simulink model "assignment_12_impedance_control_2022a"  (R2022a)
settings: Solver=VariableStepAuto  StartTime=0.0  StopTime=10  RelTol=1e-3
values from neighbouring files (symbols this model uses):
  dq0 = [0;0;0]    [assignment_10.m]    (also in assignment_11.m; assignment_12.m; assignment_13.m; assignment_6.m)
  K_env = 1000    [assignment_11.m]    (also in assignment_12.m = 100; assignment_13.m = 100)
  Kd = 100    [assignment_10.m]    (also in assignment_11.m = 1000; assignment_12.m; assignment_6.m = 1000; assignment_7.m = diag(2 * xi .* w))
  Kp = 1000    [assignment_10.m]    (also in assignment_11.m = 10000; assignment_12.m; assignment_6.m; assignment_7.m = diag(w .* w))
  q0 = [0;0;0]    [assignment_10.m]    (also in assignment_11.m; assignment_12.m; assignment_13.m = [0; pi/2; -pi/2]; assignment_6.m)
  traj = [q1_d; q2_d; q3_d]    [assignment_10.m]    (also in assignment_12.m; assignment_7.m)
  x_rest_env = direct_kinematics(q_rest_env)    [assignment_11.m]    (also in assignment_12.m; assignment_13.m = x_rest_env(1:3, 1))
libraries: robotcorelib x1
settings Model: Creator=acesi  LastModifiedBy=Manu
settings ModelReferenceCC: EnableRefExpFcnMdlSchedulingChecks=off
settings RTWCC: Description=Generic Real-Time Target

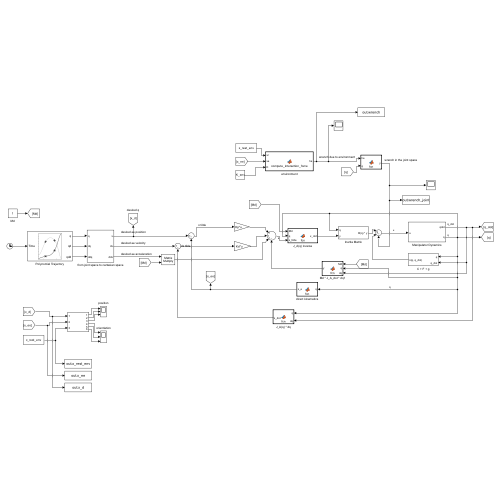
[thumbnail: Simulink's stored preview of the top-level diagram]
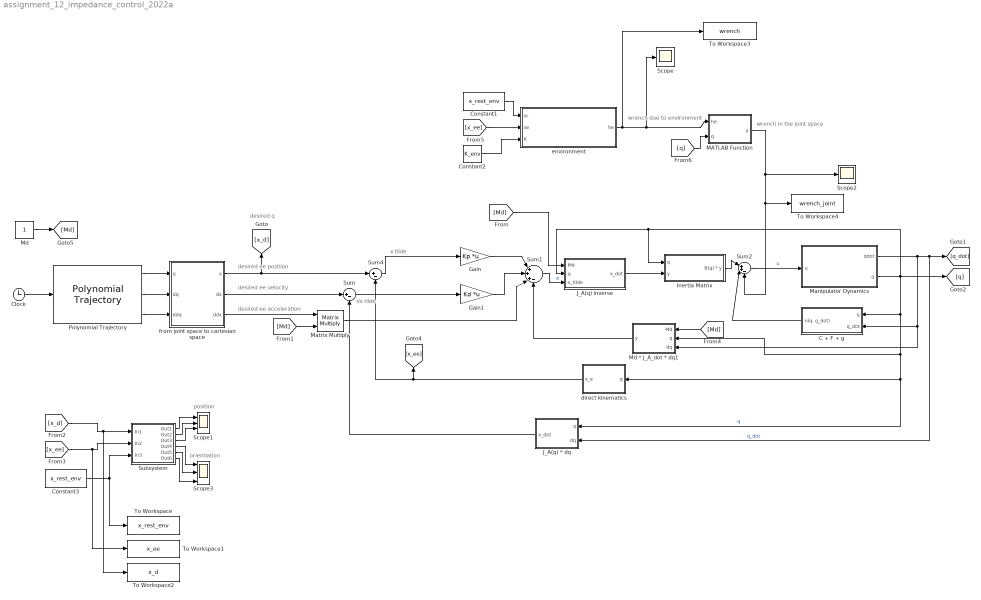
== system assignment_12_impedance_control_2022a ==
  note: x tilde
  note: desired q
  note: desired ee position
  note: desired ee acceleration
  note: dx tilde
  note: orientiation
  note: position
  note: desired ee velocity
  note: wrench due to environment
  note: wrench in the joint space
  C + F + g : Subsystem
  Clock : Clock
  Constant1 : Constant  Value=x_rest_env
  Constant2 : Constant  Value=K_env
  Constant3 : Constant  Value=x_rest_env
  Gain : Gain  Gain=Kp  Multiplication=Matrix(K*u)
  Gain1 : Gain  Gain=Kd  Multiplication=Matrix(K*u)
  Inertia Matrix : Subsystem
  J_A(q) * dq : MATLAB Function  TreatAsAtomicUnit=on
  J_A(q) inverse : MATLAB Function  TreatAsAtomicUnit=on
  MATLAB Function : MATLAB Function  TreatAsAtomicUnit=on
  Manipulator Dynamics : Subsystem
  Matrix Multiply : Product  Multiplication=Matrix(*)
  Md : Constant
  Md * J_A_dot * dq1 : MATLAB Function  TreatAsAtomicUnit=on
  Polynomial Trajectory : robotcorelib/Polynomial Trajectory  WaypointSource=Internal  Waypoints=traj  TimePoints=time_vector  TimeInterval=[ 1, 10 ]  Method=Cubic Polynomial  ParameterSource=Internal  VelocityBoundaryCondition=zeros(size(traj))  AccelerationBoundaryCondition=zeros(size(traj))  SimulateUsing=Interpreted execution
  Scope : Scope
  Scope1 : Scope  NumInputPorts=3
  Scope2 : Scope
  Scope3 : Scope  NumInputPorts=3
  Subsystem : Subsystem
  Sum : Sum  Inputs=|+-
  Sum1 : Sum  Inputs=|+++-
  Sum2 : Sum  Inputs=|++-
  Sum4 : Sum  Inputs=|+-
  To Workspace : ToWorkspace  VariableName=x_rest_env  SaveFormat=Timeseries  SampleTime=-1
  To Workspace1 : ToWorkspace  VariableName=x_ee  SaveFormat=Timeseries  SampleTime=-1
  To Workspace2 : ToWorkspace  VariableName=x_d  SaveFormat=Timeseries  SampleTime=-1
  To Workspace3 : ToWorkspace  VariableName=wrench  SaveFormat=Timeseries  SampleTime=-1
  To Workspace4 : ToWorkspace  VariableName=wrench_joint  SaveFormat=Timeseries  SampleTime=-1
  direct kinematics : MATLAB Function  TreatAsAtomicUnit=on
  environment : MATLAB Function  TreatAsAtomicUnit=on
  from joint space to cartesian space : Subsystem
  wires:
  Manipulator Dynamics/1(qdot) -> J_A(q) * dq/2(dq), [q_dot], Md * J_A_dot * dq1/3(dq), C + F + g/2(q_dot)  "q_dot"
  Manipulator Dynamics/2(q) -> Md * J_A_dot * dq1/2(q), J_A(q) * dq/1(q), direct kinematics/1(q), C + F + g/1(q), [q], J_A(q) inverse/2(q), Inertia Matrix/1(q)  "q"
  Inertia Matrix/1(B(q) * y) -> Sum2/1
  Sum2/1 -> Manipulator Dynamics/1(u)  "u"
  C + F + g/1("n(q, q_dot)") -> Sum2/2
  Clock/1 -> Polynomial Trajectory/1
  Gain/1 -> Sum1/1
  Gain1/1 -> Sum1/2
  Sum/1 -> Gain1/1
  Sum4/1 -> Gain/1
  direct kinematics/1(x_e) -> Sum4/2, [x_ee]
  J_A(q) * dq/1(x_dot) -> Sum/2
  Sum1/1 -> J_A(q) inverse/3(x_tilde)  "e"
  J_A(q) inverse/1(x_dot) -> Inertia Matrix/2(y)
  [x_d] -> Subsystem/1(In1), To Workspace2/1
  [x_ee] -> Subsystem/2(In2), To Workspace1/1
  Subsystem/6(Out6) -> Scope3/3
  Subsystem/2(Out2) -> Scope1/2
  Subsystem/4(Out4) -> Scope3/1
  Subsystem/3(Out3) -> Scope1/3
  Subsystem/5(Out5) -> Scope3/2
  Subsystem/1(Out1) -> Scope1/1
  Md * J_A_dot * dq1/1(y) -> Sum1/4
  Polynomial Trajectory/1 -> from joint space to cartesian space/1(q)
  Polynomial Trajectory/2 -> from joint space to cartesian space/2(dq)
  Polynomial Trajectory/3 -> from joint space to cartesian space/3(ddq)
  from joint space to cartesian space/3(ddx) -> Matrix Multiply/1
  from joint space to cartesian space/2(dx) -> Sum/1
  from joint space to cartesian space/1(x) -> Sum4/1, [x_d]
  [Md] -> J_A(q) inverse/1(Md)
  Md/1 -> [Md]
  [Md] -> Matrix Multiply/2
  Matrix Multiply/1 -> Sum1/3
  [Md] -> Md * J_A_dot * dq1/1(Md)
  Constant2/1 -> environment/3(K)
  [x_ee] -> environment/2(xe)
  Constant1/1 -> environment/1(xr)
  environment/1(he) -> MATLAB Function/1(he), Scope/1, To Workspace3/1
  [q] -> MATLAB Function/2(q)
  MATLAB Function/1(y) -> Scope2/1, To Workspace4/1, Sum2/3
  Constant3/1 -> To Workspace/1, Subsystem/3(In3)

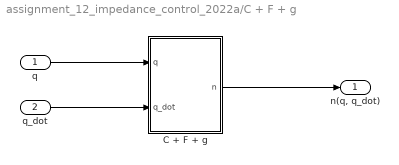
== system assignment_12_impedance_control_2022a/C + F + g ==
  q : Inport
  q_dot : Inport  Port=2
  C + F + g : MATLAB Function  TreatAsAtomicUnit=on
  "n(q, q_dot)" : Outport
  wires:
  C + F + g/1(n) -> "n(q, q_dot)"/1
  q/1 -> C + F + g/1(q)
  q_dot/1 -> C + F + g/2(q_dot)

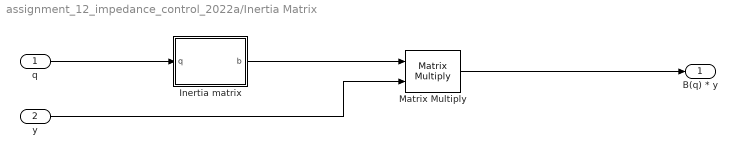
== system assignment_12_impedance_control_2022a/Inertia Matrix ==
  q : Inport
  y : Inport  Port=2
  Inertia matrix : MATLAB Function  TreatAsAtomicUnit=on
  Matrix Multiply : Product  Multiplication=Matrix(*)
  B(q) * y : Outport
  wires:
  q/1 -> Inertia matrix/1(q)
  Inertia matrix/1(b) -> Matrix Multiply/1
  y/1 -> Matrix Multiply/2
  Matrix Multiply/1 -> B(q) * y/1

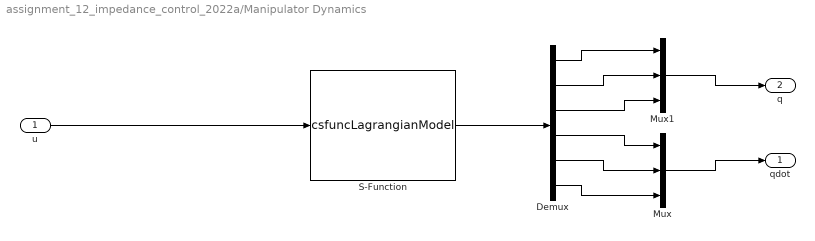
== system assignment_12_impedance_control_2022a/Manipulator Dynamics ==
  u : Inport
  Demux : Demux  Outputs=6
  Mux : Mux  Inputs=3
  Mux1 : Mux  Inputs=3
  S-Function : S-Function  FunctionName=csfuncLagrangianModel  Parameters=q0 dq0  SFunctionDeploymentMode=off  EnableBusSupport=off
  qdot : Outport
  q : Outport  Port=2
  wires:
  u/1 -> S-Function/1
  S-Function/1 -> Demux/1
  Mux1/1 -> q/1
  Mux/1 -> qdot/1
  Demux/6 -> Mux/3
  Demux/5 -> Mux/2
  Demux/4 -> Mux/1
  Demux/3 -> Mux1/3
  Demux/2 -> Mux1/2
  Demux/1 -> Mux1/1

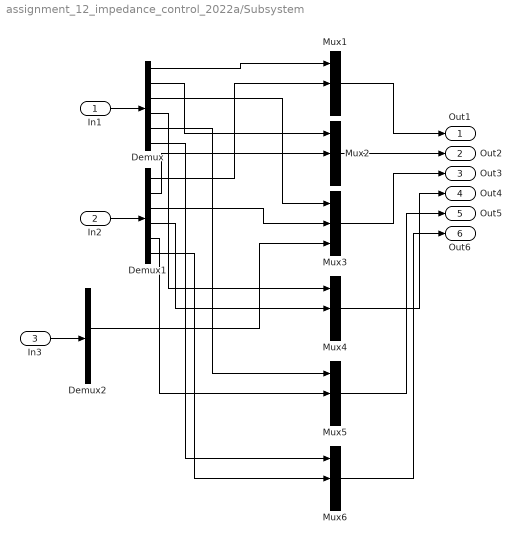
== system assignment_12_impedance_control_2022a/Subsystem ==
  In1 : Inport
  In2 : Inport  Port=2
  In3 : Inport  Port=3
  Demux : Demux  Outputs=6
  Demux1 : Demux  Outputs=6
  Demux2 : Demux  Outputs=6
  Mux{1..6} (6 alike) : Mux  Inputs=3
  Out1 : Outport
  Out2 : Outport  Port=2
  Out3 : Outport  Port=3
  Out4 : Outport  Port=4
  Out5 : Outport  Port=5
  Out6 : Outport  Port=6
  wires:
  Demux/1 -> Mux1/1
  Demux/3 -> Mux3/1
  Demux/2 -> Mux2/1
  Demux1/1 -> Mux1/2
  Mux2/1 -> Out2/1
  Demux1/3 -> Mux3/2
  Demux1/2 -> Mux2/2
  Mux3/1 -> Out3/1
  Mux1/1 -> Out1/1
  In2/1 -> Demux1/1
  In1/1 -> Demux/1
  Demux1/4 -> Mux4/2
  Demux/4 -> Mux4/1
  Demux/5 -> Mux5/1
  Demux1/5 -> Mux5/2
  Demux/6 -> Mux6/1
  Demux1/6 -> Mux6/2
  Mux4/1 -> Out4/1
  Mux5/1 -> Out5/1
  Mux6/1 -> Out6/1
  In3/1 -> Demux2/1
  Demux2/3 -> Mux3/3

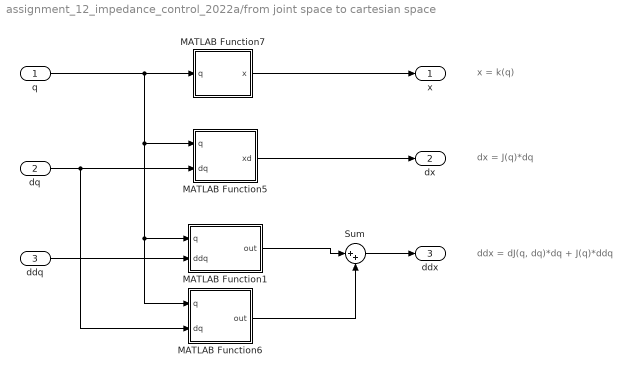
== system assignment_12_impedance_control_2022a/from joint space to cartesian space ==
  note: ddx = dJ(q, dq)*dq + J(q)*ddq
  note: dx = J(q)*dq
  note: x = k(q)
  q : Inport
  dq : Inport  Port=2
  ddq : Inport  Port=3
  MATLAB Function1 : MATLAB Function  TreatAsAtomicUnit=on
  MATLAB Function5 : MATLAB Function  TreatAsAtomicUnit=on
  MATLAB Function6 : MATLAB Function  TreatAsAtomicUnit=on
  MATLAB Function7 : MATLAB Function  TreatAsAtomicUnit=on
  Sum : Sum  Inputs=|++
  x : Outport
  dx : Outport  Port=2
  ddx : Outport  Port=3
  wires:
  q/1 -> MATLAB Function5/1(q), MATLAB Function6/1(q), MATLAB Function1/1(q), MATLAB Function7/1(q)
  MATLAB Function7/1(x) -> x/1
  MATLAB Function5/1(xd) -> dx/1
  ddq/1 -> MATLAB Function1/2(ddq)
  dq/1 -> MATLAB Function5/2(dq), MATLAB Function6/2(dq)
  MATLAB Function6/1(out) -> Sum/2
  MATLAB Function1/1(out) -> Sum/1
  Sum/1 -> ddx/1

== matlab function assignment_12_impedance_control_2022a/Inertia Matrix/Inertia matrix ==
  data: q input; b output
function b = B(q)

    b = get_B_hardcoded(q);

end

== matlab function assignment_12_impedance_control_2022a/C + F + g/C + F + g ==
  data: q input; n output; q_dot input
function n = N(q, q_dot)
    % return n = C(q, qd) + F + g(q) 

    g = get_G_hardcoded(q);
    c = get_C_hardcoded(q, q_dot) * q_dot;

    n = g + c;
end

== matlab function assignment_12_impedance_control_2022a/direct kinematics ==
  data: q input; x_e output
function x_e = fcn(q)
    x_e = direct_kinematics(q);
end

== matlab function assignment_12_impedance_control_2022a/J_A(q) * dq ==
  data: q input; x_dot output; dq input
function x_dot = fcn(q, dq)
    x_dot = get_JA(q) * dq;
end

== matlab function assignment_12_impedance_control_2022a/J_A(q) inverse ==
  data: Md input; q input; x_dot output; x_tilde input
function x_dot = fcn(Md, q, x_tilde)
    x_dot = pinv(get_JA(q)) * pinv(Md) * x_tilde;
end

== matlab function assignment_12_impedance_control_2022a/MATLAB Function ==
  data: he input; y output; q input
function y = fcn(he, q)
% maps wrench to joint space (qual'è la nomenclatura corretta?)
y = get_JG(q)' * he;

== matlab function assignment_12_impedance_control_2022a/Md * J_A_dot * dq1 ==
  data: Md input; q input; y output; dq input
function y = fcn(Md, q, dq)
    J_A_dot = get_JA_dot(q, dq);
    y = Md * J_A_dot * dq;
end

== matlab function assignment_12_impedance_control_2022a/from joint space to cartesian space/MATLAB Function7 ==
  data: q input; x output
function x = fun(q)
    x = direct_kinematics(q);
end

== matlab function assignment_12_impedance_control_2022a/from joint space to cartesian space/MATLAB Function5 ==
  data: q input; dq input; xd output
function xd = fun(q, dq)
    Ja = get_JA(q);
    xd = Ja * dq;
end

== matlab function assignment_12_impedance_control_2022a/from joint space to cartesian space/MATLAB Function1 ==
  data: q input; ddq input; out output
function out = fun(q, ddq)
    Ja = get_JA(q);
    out = Ja * ddq;
end

== matlab function assignment_12_impedance_control_2022a/from joint space to cartesian space/MATLAB Function6 ==
  data: q input; dq input; out output
function out = fun(q, dq)
    d_Ja = get_JA_dot(q,dq);
    out = d_Ja * dq;
end

== matlab function assignment_12_impedance_control_2022a/environment ==
  data: xr input; he output; xe input; K input
function he = compute_interaction_force(xr, xe, K)
% xr: rest position of the environment (expressed in the operational space)
% xe: current position of the end effector (expressed in the operational space)
% K: environment spring constant (the env. is modeled as a pure spring)

if xe(3) < xr(3)
    he = zeros(6,1); % no interaction with the environment
else
    % end effector position is larger than the env. rest position
    delta_position = xr - xe;
    he = -K * delta_position; % spring force: f = -kx

    % simulate force only on the z-axis
    he(1:2, 1) = 0; % set x, y components to 0
    he(4:6, 1) = 0; % set orientation components to 0
end
